simulink model "Slip_Calculation"  (R2023b)
settings: Solver=FixedStepDiscrete  StartTime=0.0  StopTime=10.0  FixedStep=0.01  RelTol=1e-3
settings Model: Creator=E8KUAVE  LastModifiedBy=E8KUAVE
settings DataIOCC: ExternalInput=[100 100 100], [80 90 70]  LoadExternalInput=on
settings OptimizationCC: DefaultParameterBehavior=Inlined  EnhancedBackFolding=on  PassReuseOutputArgsAs=Individual arguments  ZeroExternalMemoryAtStartup=off  ZeroInternalMemoryAtStartup=off  OptimizeBlockOrder=speed  DifferentSizesBufferReuse=on  OptimizationCustomize=off  EfficientTunableParamExpr=on
settings DebuggingCC: ParameterTunabilityLossMsg=error
settings HardwareCC: ProdBitPerPointer=32  ProdBitPerSizeT=32  ProdBitPerPtrDiffT=32  ProdLargestAtomicInteger=Long  ProdLargestAtomicFloat=Double  ProdWordSize=32  ProdHWDeviceType=ARM Compatible->ARM Cortex-M
settings SFSimCC: MATLABDynamicMemAlloc=off  SimTargetLang=C++
settings RTWCC: Description=Embedded Coder  SystemTargetFile=ert.tlc  GenCodeOnly=on  TemplateMakefile=ert_default_tmf  Toolchain=MinGW64 | gmake (64-bit Windows)  DataTypeReplacement=CDataTypesFixedWidth  TargetLang=C++
settings CodeAppCC: ForceParamTrailComments=on  IgnoreCustomStorageClasses=off  OperatorAnnotations=on  SimulinkDataObjDesc=on  SFDataObjDesc=on  InsertBlockDesc=on
settings ERTTargetCC: TargetLangStandard=C++11 (ISO)  GenerateSampleERTMain=on  CodeInterfacePackaging=C++ class  PurelyIntegerCode=on  SupportNonFinite=off  InlinedParameterPlacement=NonHierarchical  RootIOFormat=Structure reference  ERTCustomFileTemplate=example_file_process.tlc  MaxIdInt64=INT64_MAX  MinIdInt64=INT64_MIN  MaxIdUint64=UINT64_MAX  MaxIdInt32=INT32_MAX  MinIdInt32=INT32_MIN  MaxIdUint32=UINT32_MAX  MaxIdInt16=INT16_MAX  MinIdInt16=INT16_MIN  MaxIdUint16=UINT16_MAX  MaxIdInt8=INT8_MAX  MinIdInt8=INT8_MIN  MaxIdUint8=UINT8_MAX

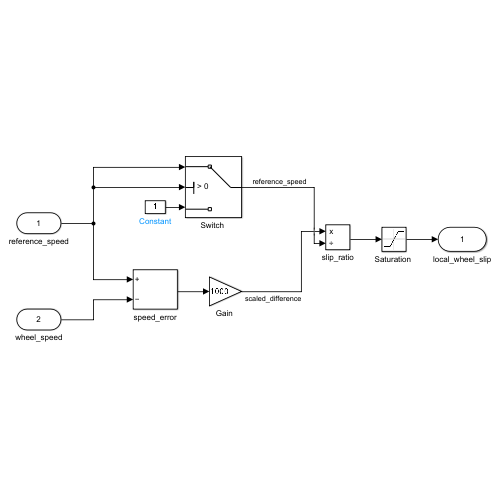
[thumbnail: Simulink's stored preview of the top-level diagram]
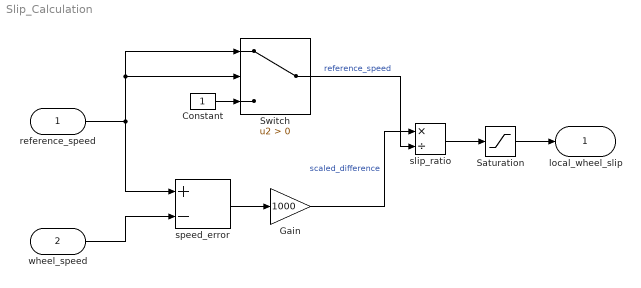
== system Slip_Calculation ==
  reference_speed : Inport  OutDataTypeStr=uint16
  wheel_speed : Inport  Port=2  OutDataTypeStr=uint16
  Constant : Constant  OutDataTypeStr=int16
  "Gain " : Gain  Gain=1000  OutDataTypeStr=int32
  "Saturation " : Saturate  UpperLimit=1000  LowerLimit=0  OutDataTypeStr=uint16
  "Switch " : Switch  Criteria=u2 > Threshold  SaturateOnIntegerOverflow=off  InputSameDT=off
  slip_ratio : Product  Inputs=*/  OutDataTypeStr=int32
  speed_error : Sum  Inputs=+-  OutDataTypeStr=int32
  local_wheel_slip : Outport  OutDataTypeStr=uint16
  wires:
  reference_speed/1 -> speed_error/1, "Switch "/1, "Switch "/2
  wheel_speed/1 -> speed_error/2
  speed_error/1 -> "Gain "/1
  "Gain "/1 -> slip_ratio/1  "scaled_difference"
  slip_ratio/1 -> "Saturation "/1
  "Saturation "/1 -> local_wheel_slip/1
  Constant/1 -> "Switch "/3
  "Switch "/1 -> slip_ratio/2  "reference_speed"
